simulink model "BUCK_BOOST_PE_IDEAL"  (R2024a)
settings: Solver=VariableStepAuto  StartTime=0.0  StopTime=10.0  RelTol=1e-3
undefined symbols (not defined in the file): Ts
libraries: spsRMSLib x5, spsMeanLib x4, spsCurrentMeasurementLib x3, spsSeriesRLCBranchLib x3, spsGroundLib x2, spsVoltageMeasurementLib x2, spsDCVoltageSourceLib x1, spsDiodeLib x1, spsMosfetLib x1, spsPWMGeneratorDCDCLib x1, sps_lib x1
settings Model: Creator=himes  LastModifiedBy=himes
settings SolverCC: ZeroCrossAlgorithm=Adaptive
settings DebuggingCC: IgnoredZcDiagnostic=none

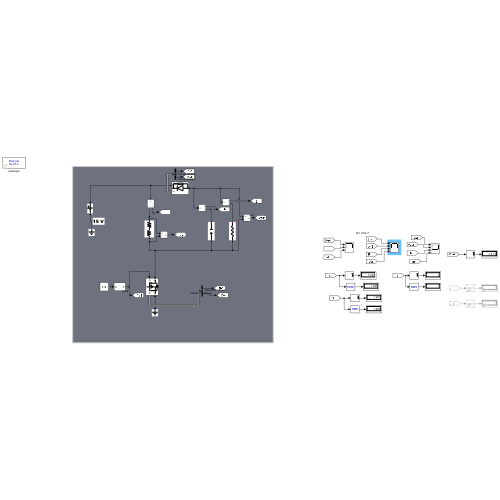
[thumbnail: Simulink's stored preview of the top-level diagram]
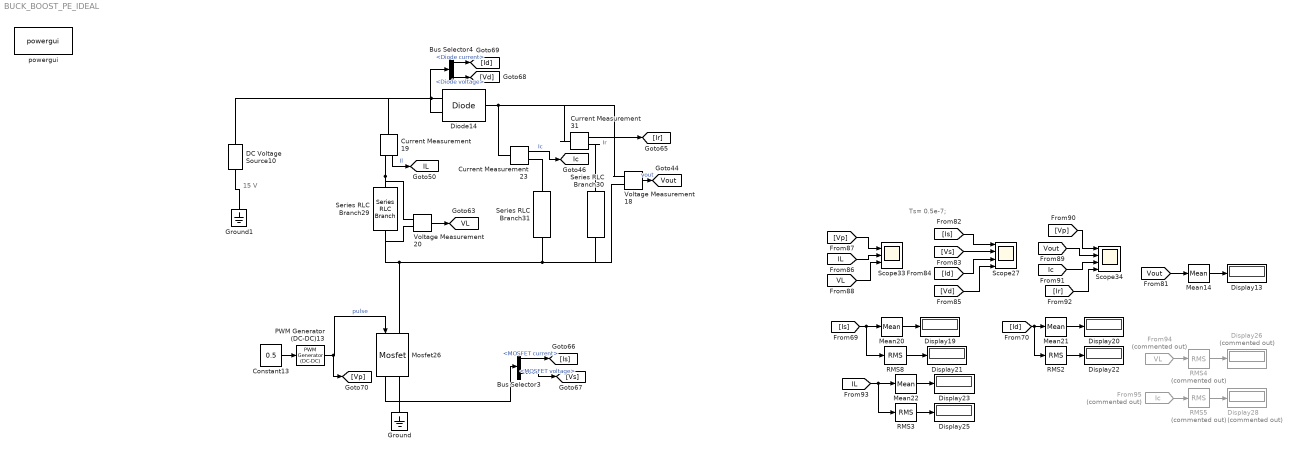
== system BUCK_BOOST_PE_IDEAL ==
  note: 15 V
  note: Ts= 0.5e-7;
  Bus Selector3 : BusSelector  OutputSignals=MOSFET current,MOSFET voltage
  Bus Selector4 : BusSelector  OutputSignals=Diode current,Diode voltage
  Constant13 : Constant  Value=0.5
  Current Measurement19 : spsCurrentMeasurementLib/Current Measurement  PhasorSimulation=off  OutputType=Complex  PSBequivalent=0
  Current Measurement23 : spsCurrentMeasurementLib/Current Measurement  PhasorSimulation=off  OutputType=Complex  PSBequivalent=0
  Current Measurement31 : spsCurrentMeasurementLib/Current Measurement  PhasorSimulation=off  OutputType=Complex  PSBequivalent=0
  DC Voltage Source10 : spsDCVoltageSourceLib/DC Voltage Source  Amplitude=15  Measurements=None
  Diode14 : spsDiodeLib/Diode  Ron=0.15  Lon=0  Vf=1.75  IC=0  UseSnubber=0  Rs=1e6  Cs=1e6  Measurements=on
  Display{13,19..23,25} (7 alike) : Display
  Display26 : Display  Commented=on
  Display28 : Display  Commented=on
  From94 : From  Commented=on  GotoTag=VL  TagVisibility=global
  From95 : From  Commented=on  GotoTag=Ic  TagVisibility=global
  Ground : spsGroundLib/Ground  LConnTagsString=a
  Ground1 : spsGroundLib/Ground  LConnTagsString=a
  Mean{14,20..22} (4 alike) : spsMeanLib/Mean  Freq=50000  Vinit=0  Ts=0
  Mosfet26 : spsMosfetLib/Mosfet  Ron=1e-7  Lon=0  Rd=0.022  Vfd=0  IC=0  Rs=inf  Cs=0  Measurements=on
  PWM Generator (DC-DC)13 : spsPWMGeneratorDCDCLib/PWM Generator (DC-DC)  Fsw=12500  Ts=Ts
  RMS2 : spsRMSLib/RMS  TrueRMS=on  Freq=50000  RMSInit=0  Ts=0
  RMS3 : spsRMSLib/RMS  TrueRMS=on  Freq=50000  RMSInit=0  Ts=0
  RMS4 : spsRMSLib/RMS  Commented=on  TrueRMS=on  Freq=50000  RMSInit=0  Ts=0
  RMS5 : spsRMSLib/RMS  Commented=on  TrueRMS=on  Freq=50000  RMSInit=0  Ts=0
  RMS8 : spsRMSLib/RMS  TrueRMS=on  Freq=50000  RMSInit=0  Ts=0
  Scope27 : Scope  NumInputPorts=4
  Scope33 : Scope  NumInputPorts=3
  Scope34 : Scope  NumInputPorts=4
  Series RLC Branch29 : spsSeriesRLCBranchLib/Series RLC Branch  LConnTagsString=__new0  RConnTagsString=__new0  BranchType=RL  Resistance=0.4  Inductance=0.001  SetiL0=off  InitialCurrent=0  Capacitance=1e-6  Setx0=off  InitialVoltage=0  Measurements=None
  Series RLC Branch30 : spsSeriesRLCBranchLib/Series RLC Branch  LConnTagsString=__new0  RConnTagsString=__new0  BranchType=R  Resistance=16  Inductance=1e-3  SetiL0=off  InitialCurrent=0  Capacitance=1000e-6  Setx0=on  InitialVoltage=800  Measurements=None
  Series RLC Branch31 : spsSeriesRLCBranchLib/Series RLC Branch  LConnTagsString=__new0  RConnTagsString=__new0  BranchType=C  Resistance=6  Inductance=1e-3  SetiL0=off  InitialCurrent=0  Capacitance=200e-6  Setx0=off  InitialVoltage=800  Measurements=None
  Voltage Measurement18 : spsVoltageMeasurementLib/Voltage Measurement  PhasorSimulation=off  OutputType=Complex  PSBequivalent=0
  Voltage Measurement20 : spsVoltageMeasurementLib/Voltage Measurement  PhasorSimulation=off  OutputType=Complex  PSBequivalent=0
  powergui : sps_lib/powergui  Priority=1  SimulationMode=Discrete  SampleTime=Ts  frequency=60  Iterations=50  frequencyindice=0  Pbase=100e6  ErrMax=1e-4  UnitsV=kV  UnitsW=MW  buscounter=0  FunctionMessages=off  echomessages=off  EnableUseOfTLC=off  CurrentSourceSwitches=off  DisableSnubberDevices=off  DisableRonSwitches=off  DisableVfSwitches=off  DisplayEquations=off  AutomaticDiscreteSolvers=off  SolverType=Tustin/Backward Euler (TBE)  Interpol=off  ExternalGateDelay=off  methode=off  Ts=100  x0status=blocks  SPID=on  SwTol=0  HookPort=off  NonlinearTolerance=1e-4  nMaxIteration=100  ContinueOnMaxIteration=off  RestoreLinks=warning  ResistiveCurrentMeasurement=off  Frange=[0:2:500]  Ylog=off  Xlog=on  ShowGrid=off  save=off  variable=ZData  structure=0  ZoomFFT=off  StartTime=0.0  cycles=1  DisplayStyle=1  fundamental=60  FreqAxis=off  MaxFrequency=1000  frequencyindicesteady=1  RmsSteady=1  display=off
  tag scope: IL=global, Ic=global, VL=global, Vout=global
  wires:
  Current Measurement23/1 -> [Ic]  "Ic"
  Diode14/1 -> Bus Selector4/1
  Current Measurement31/1 -> [Ir]  "Ir"
  Bus Selector4/2 -> [Vd]  "<Diode voltage>"
  Bus Selector4/1 -> [Id]  "<Diode current>"
  Voltage Measurement20/1 -> [VL]
  Current Measurement19/1 -> [IL]  "Il"
  Voltage Measurement18/1 -> [Vout]  "vout"
  [Vp] -> Scope33/1
  Mean20/1 -> Display19/1
  From94/1 -> RMS4/1
  [Vs] -> Scope27/2
  RMS3/1 -> Display25/1
  From95/1 -> RMS5/1
  [Ic] -> Scope34/3
  [Is] -> Scope27/1
  Mean14/1 -> Display13/1
  [Id] -> Scope27/3
  [Vd] -> Scope27/4
  [Ir] -> Scope34/4
  RMS5/1 -> Display28/1
  Mean21/1 -> Display20/1
  [VL] -> Scope33/3
  [Vp] -> Scope34/1
  RMS4/1 -> Display26/1
  [Id] -> RMS2/1, Mean21/1
  [Is] -> RMS8/1, Mean20/1
  Mean22/1 -> Display23/1
  [IL] -> RMS3/1, Mean22/1
  [IL] -> Scope33/2
  RMS8/1 -> Display21/1
  [Vout] -> Mean14/1
  [Vout] -> Scope34/2
  RMS2/1 -> Display22/1
  Constant13/1 -> PWM Generator (DC-DC)13/1
  PWM Generator (DC-DC)13/1 -> Mosfet26/1, [Vp]  "pulse"
  Bus Selector3/1 -> [Is]  "<MOSFET current>"
  Bus Selector3/2 -> [Vs]  "<MOSFET voltage>"
  Mosfet26/1 -> Bus Selector3/1
  connections:
  Series RLC Branch29/LConn1 -- Current Measurement19/RConn1 -- Voltage Measurement20/LConn1
  Diode14/LConn1 -- Voltage Measurement18/LConn1 -- Current Measurement31/LConn1 -- Current Measurement23/LConn1
  Series RLC Branch31/RConn1 -- Voltage Measurement18/LConn2 -- Series RLC Branch30/RConn1 -- Series RLC Branch29/RConn1 -- Voltage Measurement20/LConn2 -- Mosfet26/LConn1
  Series RLC Branch31/LConn1 -- Current Measurement23/RConn1
  Diode14/RConn1 -- DC Voltage Source10/RConn1 -- Current Measurement19/LConn1
  Current Measurement31/RConn1 -- Series RLC Branch30/LConn1
  Ground/LConn1 -- Mosfet26/RConn1
  Ground1/LConn1 -- DC Voltage Source10/LConn1
